simulink model "lqr_ss"  (R2024b)
settings: Solver=VariableStepAuto  StartTime=0.0  StopTime=10.0  RelTol=1e-3
undefined symbols (not defined in the file): A_mat, B_mat, C_mat, k
settings Model: Creator=Ahmed  LastModifiedBy=Eng Abdullah Sherif
settings SolverCC: AlgebraicLoopSolver=TrustRegion
settings DebuggingCC: ArithmeticOperatorsInVariantConditions=warning
settings SFSimCC: CustomCodeUndefinedFunction=UseInterfaceOnly
settings RTWCC: GPUComputeCapability=3.5

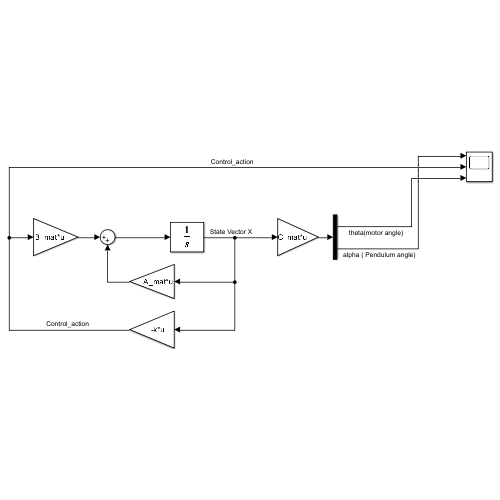
[thumbnail: Simulink's stored preview of the top-level diagram]
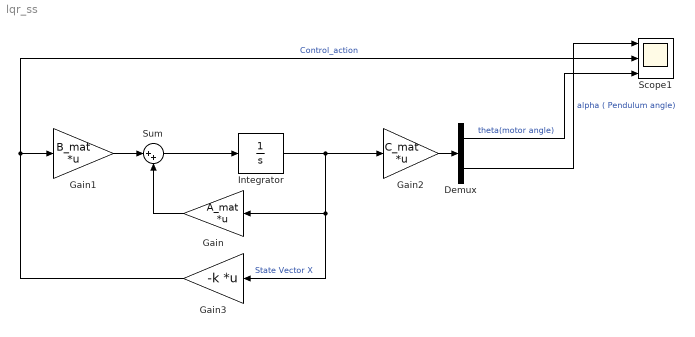
== system lqr_ss ==
  Demux : Demux  Outputs=2
  Gain : Gain  Gain=A_mat  Multiplication=Matrix(K*u)
  Gain1 : Gain  Gain=B_mat  Multiplication=Matrix(K*u)
  Gain2 : Gain  Gain=C_mat  Multiplication=Matrix(K*u)
  Gain3 : Gain  Gain=-k  Multiplication=Matrix(K*u)
  Integrator : Integrator  InitialCondition=[0.5 0.436 0 0]
  Scope1 : Scope  NumInputPorts=3
  Sum : Sum  Inputs=|++
  wires:
  Gain1/1 -> Sum/1
  Gain/1 -> Sum/2
  Sum/1 -> Integrator/1
  Gain3/1 -> Scope1/2, Gain1/1  "Control_action"
  Gain2/1 -> Demux/1
  Integrator/1 -> Gain/1, Gain3/1, Gain2/1  "State Vector X"
  Demux/2 -> Scope1/1  "alpha ( Pendulum angle)"
  Demux/1 -> Scope1/3  "theta(motor angle)"
